simulink model "relojoaria_model"  (R2018a)
settings: Solver=VariableStepAuto  StartTime=0.0  StopTime=ttotal  RelTol=1e-3  EnableMultiTasking=on
values from neighbouring files (symbols this model uses):
  beta = 0.001    [e_13.m]    (also in e_8.m = 1; e_9.m; lab3.m; lab3_1.m = 1)
  g = 9.8    [e_13.m]    (also in e_8.m; e_9.m; lab3.m; lab3_1.m)
  J = ((M*L^2)/3) + (m * l(n)^2)    [e_12.m]    (also in e_13.m = M*L^2/3+m_s*l^2; e_8.m = 0.0445; e_9.m = ((M*L^2)/3) + (m * l^2); lab3.m = M*L^2/3+m_s*l^2)
  k = 0.35    [e_13.m]    (also in e_8.m = 3; e_9.m; lab3.m; lab3_1.m = 3)
  L = 0.25    [e_13.m]    (also in e_8.m = 0.5; e_9.m; lab3.m; lab3_1.m = 0.5)
  l = l_c_nl(n)    [e_10.m]    (also in e_11.m = l_c(2); e_12.m = l_c; e_13.m = l_c(1); e_8.m = 0.4)
  M = 0.1    [e_13.m]    (also in e_8.m = 0.15; e_9.m; lab3.m; lab3_1.m = 0.15)
  m = 0.2    [e_8.m]    (also in e_9.m = m_c; lab3.m = m_c; lab3_1.m; lab3_2.m = m_c)
  T = T_v(n)    [e_11.m]    (also in e_13.m = 0; e_8.m = 0; e_9.m = 0; lab3.m = 0)
  threshold_v = 0.1    [e_11.m]    (also in lab3.m; lab3_2.m)
  x0 = [pi/4 0]    [e_13.m]    (also in e_8.m = vec_prop(:,n); e_9.m; lab3.m; lab3_1.m = [0 pi/4])
settings Model: Creator=ricar  LastModifiedBy=root
settings OptimizationCC: LifeSpan=inf
settings DebuggingCC: SFUnexpectedBacktrackingDiag=warning  SFNoUnconditionalDefaultTransitionDiag=warning  SFExecutionAtInitializationDiag=none
settings CodeAppCC: StateflowObjectComments=on
settings GRTTargetCC: TargetLangStandard=C89/C90 (ANSI)  GeneratePreprocessorConditionals=Disable all
settings ConfigComp: CovMetricSettings=dw  CovHtmlReporting=on  CovSaveCumulativeToWorkspaceVar=on  CovSaveSingleToWorkspaceVar=on  CovExternalEMLEnable=off

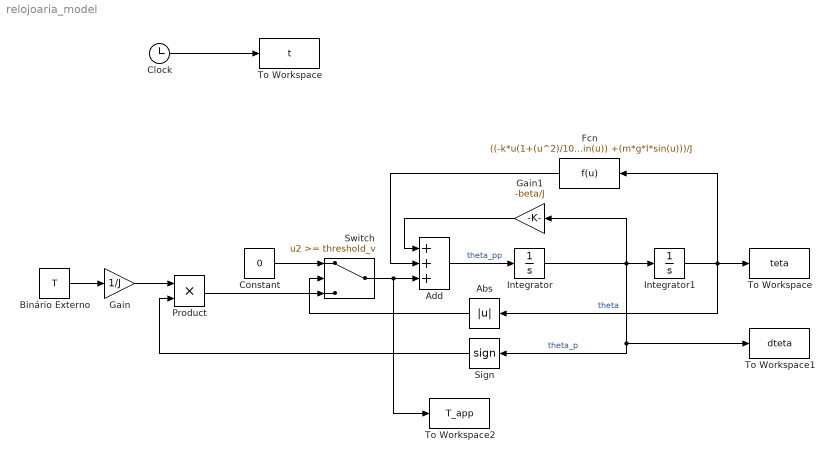
== system relojoaria_model ==
  Abs : Abs
  Add : Sum  Inputs=+++
  Binário Externo : Constant  Value=T
  Clock : Clock
  Constant : Constant  Value=0
  Fcn : Fcn  Expr=((-k*u(1+(u^2)/100))+(M*g*(L/2)*sin(u)) +(m*g*l*sin(u)))/J
  Gain : Gain  Gain=1/J
  Gain1 : Gain  Gain=-beta/J
  Integrator : Integrator  InitialCondition=x0(2)
  Integrator1 : Integrator  InitialCondition=x0(1)
  Product : Product
  Sign : Signum
  Switch : Switch  Threshold=threshold_v
  To Workspace : ToWorkspace  VariableName=teta  SampleTime=-1
  "To Workspace " : ToWorkspace  VariableName=t  SampleTime=-1
  To Workspace1 : ToWorkspace  VariableName=dteta  SampleTime=-1
  To Workspace2 : ToWorkspace  VariableName=T_app  SampleTime=-1
  wires:
  Binário Externo/1 -> Gain/1
  Add/1 -> Integrator/1  "theta_pp"
  Integrator/1 -> Gain1/1, Sign/1, To Workspace1/1, Integrator1/1  "theta_p"
  Integrator1/1 -> Abs/1, Fcn/1, To Workspace/1  "theta"
  Gain1/1 -> Add/1
  Fcn/1 -> Add/2
  Switch/1 -> To Workspace2/1, Add/3
  Constant/1 -> Switch/1
  Gain/1 -> Product/1
  Product/1 -> Switch/3
  Abs/1 -> Switch/2
  Sign/1 -> Product/2
  Clock/1 -> "To Workspace "/1
